simulink model "cell_station_2017_327_constant_load_for_battery_limit_suc"  (R2016b)
settings: Solver=VariableStepAuto  StartTime=0.0  StopTime=120*2  FixedStep=1e-6  RelTol=1e-3
undefined symbols (not defined in the file or in its folder): Acid, Lead, magnitude
libraries: powerlib x33, simulink x16, electricdrivelib x1
(part 2 of 2)

== matlab function cell_station_2017_327_constant_load_for_battery_limit_suc/Sub station 2/Controller 1/Adaptive game solver/game solver/MATLAB game1 ==
  data: E input; deadload output; deadloadold input; decaytime input; decayfactor input
function deadload  = decay(E,deadloadold,decaytime,decayfactor)
deadload=deadloadold;
power=E;
if power>100
    deadload=power;
elseif power<-100
    deadload=power;
elseif power+deadload>100||power+deadload<-100
    deadload=deadloadold;
else
    deadload=deadloadold*exp(decayfactor*decaytime);
end
end

== matlab function cell_station_2017_327_constant_load_for_battery_limit_suc/Sub station 2/Controller 1/Adaptive game solver/game solver/MATLAB game2 ==
  data: k output; SoC input; ti input; b0 input; phi input; label input; t_int input; alphao output; Energy input; deadloadold input; E input
function [k, alphao]  = multipleload(SoC,ti,b0,phi,label,t_int,Energy,deadloadold,E)
t=ti;
wa=1-b0;
amin=1;
batterystage=100;
daygoal=0.8;
sitenumber=3;
rate=[0.1 0.4 0.5];
operation=[1,1,1];
p0=10;
k=0;
power=E;
deadload=deadloadold;
% if power>120
%     deadload=power-120;
% elseif power<-120
%     deadload=power+120;
% else
%     deadload=deadloadold;
% end
[~, ~,alphao, k]=gamesolver_virtual_load_sinmulink(label,t_int,SoC,t,wa,b0,batterystage,Energy,amin,daygoal,phi,sitenumber,rate,operation,deadload);
end

== matlab function cell_station_2017_327_constant_load_for_battery_limit_suc/Sub station 1/Controller 1/Adaptive game solver/game solver/MATLAB game2 ==
  data: k output; SoC input; ti input; b0 input; phi input; label input; t_int input; alphao output; Energy input; deadloadold input; E input
function [k, alphao]  = multipleload(SoC,ti,b0,phi,label,t_int,Energy,deadloadold,E)
t=ti;
wa=1-b0;
amin=1;
batterystage=100;
daygoal=0.8;
sitenumber=3;
rate=[0.1 0.4 0.5];
operation=[1,1,1];
p0=10;
k=0;
power=E;
deadload=deadloadold;
% if power>120
%     deadload=power-120;
% elseif power<-120
%     deadload=power+120;
% else
%     deadload=deadloadold;
% end
[~, ~,alphao, k]=gamesolver_virtual_load_sinmulink(label,t_int,SoC,t,wa,b0,batterystage,Energy,amin,daygoal,phi,sitenumber,rate,operation,deadload);
end

== matlab function cell_station_2017_327_constant_load_for_battery_limit_suc/Sub station 3/Controller 1/Adaptive game solver/MATLAB game1 ==
  data: ti input; sitaguess output; phi input; label input; SoC input; SoC_old input; E output; alphao input; kself input; Estar output; sampletime input; E_aux input; Energy input
function [sitaguess,E,Estar] = multipleload(ti,phi,label,SoC,SoC_old,alphao,kself,sampletime,E_aux,Energy)
if SoC_old>0.1
p0=10;
t=ti/5;
rate=[0.1 0.4 0.5];

E=load2nojump(t)*rate(label)*kself+load2nojump(t)*(1-rate(label))*alphao(label)-solarnojump(t)*(solarnojump(t)>0)+p0*phi;
% sampletime=0.2;
% Estar=-(SoC-SoC_old)*Energy/sampletime;
Estar=-E_aux*Energy;
if abs(Estar)>48*360
    Estar=0;
end
 e0=E-Estar;
% e0=E-po;
sitaguess=0.5e-1*(e0*p0);
else
sitaguess=0;
E=0;
Estar=0;
e0=0;
end
end
%  
% function Pload=load2nojump(t)
% pl1 =    0.000839 ;
% pl2 =       1.205  ;
% pl3 =      -12.02 ;
% pl4 =       34.29  ;
% ql1 =      -6.495  ;
% ql2 =       43.45  ;
% Pload =max(0,(30* (pl1*(t).^3 + pl2*(t).^2 + pl3*(t) + pl4) ./((t).^2 + ql1*(t) + ql2))*(1+(0.2*rand-0.2*rand)*0));
% end


% 
% function [ko,koreal,alphao, kself] = gamesolver_virtual_load2(t_int,v,t,~,b0,batterystage,Energy,amin,daygoal,phi,sitenumber,rate,operation)
% alphao=zeros(1,sitenumber);
% kself=zeros(1,sitenumber);
% SoC=(v-56)*0.05+0.5;
% daygoal2=daygoal*batterystage;
% T=1;
% n=20;
% dT=T/n;
% realp=zeros(1,9);
% coder.extrinsic('linearprograming')
% coder.varsize('cost1','cost2','realrow','realcolumn')
% decide=zeros(1,sitenumber);
% P=zeros(1,batterystage*1.5);
% p=zeros(1,9);
% po=zeros(1,9);
% for ppt=1:sitenumber
%     if operation(ppt)~=0
%     opteva=zeros(9);
%     cost1=zeros(9);  
%     loadrate=rate(ppt);
% for k0=amin:1:9
%  for sigmaother0=amin:1:9
%         k=k0*0.1;
%         sigmaother=sigmaother0*0.1;       
%         [En,Sn]=pdf2_virtual_load(t,dT,loadrate,k,sigmaother,n*(24-t_int),phi(ppt));
%         if t_int~=24
%         for l=1:(batterystage*1.5)
%         P(l)=normcdf(((Energy/batterystage*(l+1)-SoC*Energy)-En*(24-t_int))/sqrt(Sn))-(normcdf(((Energy/batterystage*(l)-SoC*Energy)-En*(24-t_int))/sqrt(Sn)));
%         end
%         if (1-sum(P(1:daygoal2)))>0.5 %if there is  possibility reaching 0.8 SoC?
%             opteva(k0,sigmaother0)=b0*(sum(P(daygoal2:end)));
%             cost1(k0,sigmaother0)=((k*loadrate+sigmaother*(1-loadrate))*(1-b0)*SoC+opteva(k0,sigmaother0));
%         else  %if not stay at minimum alpha
%             cost1(k0,sigmaother0)=(1-k)/10;
%         end
%         else
%             cost1(k0,sigmaother0)=(k*loadrate+sigmaother*(1-loadrate))*(1-b0)+b0*SoC;
%         end
%  end
% end
%  [m,~]=size(cost1);
%  realrow=1:m;
% p(1:amin-1)=0;
% p(amin:9)=linearprograming(cost1(amin:9,amin:9))';
% po(1:amin-1)=0;
% po(amin:9)=linearprograming(cost1(amin:9,amin:9)')';
% linespace=0.1:0.1:0.9;
% alphao(ppt)=po*linespace';
% realn=size(realrow,2);
% for i=1:realn    
%     realp(realrow(i))=p(i);
% end
% r=rand;
% l=0;
% for i=1:9        
%     l=l+realp(i);
%     if l>r
%         break
%     end
% end
% decide(ppt)=i*0.1; 
%     end
% end
% kself=decide;
% ko=decide*rate(1:sitenumber)'/sum(rate(1:sitenumber));
% koreal=decide*rate(1:sitenumber)';
% end

== matlab function cell_station_2017_327_constant_load_for_battery_limit_suc/Sub station 3/Controller 1/Adaptive game solver/game solver/MATLAB game1 ==
  data: E input; deadload output; deadloadold input; decaytime input; decayfactor input
function deadload  = decay(E,deadloadold,decaytime,decayfactor)
deadload=deadloadold;
power=E;
if power>100
    deadload=power;
elseif power<-100
    deadload=power;
elseif power+deadload>100||power+deadload<-100
    deadload=deadloadold;
else
    deadload=deadloadold*exp(decayfactor*decaytime);
end
end

== matlab function cell_station_2017_327_constant_load_for_battery_limit_suc/Sub station 3/Controller 1/Adaptive game solver/game solver/MATLAB game2 ==
  data: k output; SoC input; ti input; b0 input; phi input; label input; t_int input; alphao output; Energy input; deadloadold input; E input
function [k, alphao]  = multipleload(SoC,ti,b0,phi,label,t_int,Energy,deadloadold,E)
t=ti;
wa=1-b0;
amin=1;
batterystage=100;
daygoal=0.8;
sitenumber=3;
rate=[0.1 0.4 0.5];
operation=[1,1,1];
p0=10;
k=0;
power=E;
deadload=deadloadold;
% if power>120
%     deadload=power-120;
% elseif power<-120
%     deadload=power+120;
% else
%     deadload=deadloadold;
% end
[~, ~,alphao, k]=gamesolver_virtual_load_sinmulink(label,t_int,SoC,t,wa,b0,batterystage,Energy,amin,daygoal,phi,sitenumber,rate,operation,deadload);
end
